simulink model "three_phase_full_bridge_rectification_mode"  (R2020b)
settings: Solver=VariableStepAuto  StartTime=0.0  StopTime=0.1  MaxStep=1e-3  RelTol=1e-3
libraries: powerlib x13, powerlib_meascontrol x4
settings Model: Creator=海王星之矛  LastModifiedBy=海王星之矛

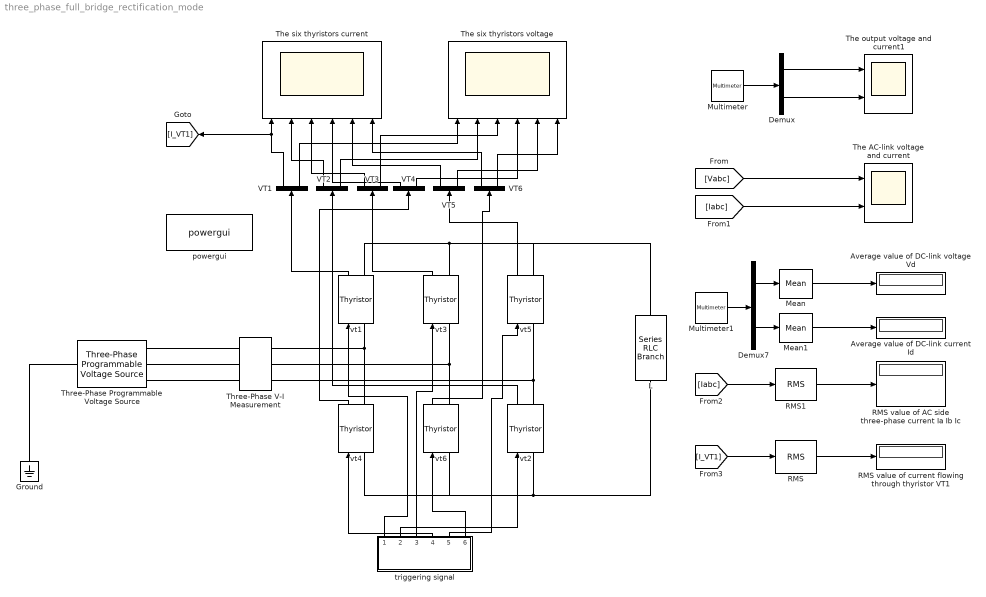
== system three_phase_full_bridge_rectification_mode ==
  Average value of DC-link current Id : Display
      settings: Decimation=2
  Average value of DC-link voltage Vd : Display
      settings: Decimation=2
  Demux : Demux  Outputs=2
  Demux7 : Demux  Outputs=2
  Ground : powerlib/Elements/Ground  LConnTagsString=a
  L : powerlib/Elements/Series RLC Branch  LConnTagsString=__new0  RConnTagsString=__new0  BranchType=RL  Resistance=1  Inductance=5e-3  SetiL0=on  InitialCurrent=0  Capacitance=1e-6  Setx0=off  InitialVoltage=0  Measurements=Branch voltage and current
  Mean : powerlib_meascontrol/Measurements/Mean  Freq=50  Vinit=0  Ts=0
  Mean1 : powerlib_meascontrol/Measurements/Mean  Freq=50  Vinit=0  Ts=0
  Multimeter : powerlib/Measurements/Multimeter  PhasorSimulation=off  OutputType=Complex  sel=[1 2]  L=2  Gain=[1 1]  yselected={'Ub: L','Ib: L'};  PSBOutputType=1  PSBequivalent=0  AxesSetting=[0,0.1,-100,100]  Display=0  SavedBlockNames=-11
  Multimeter1 : powerlib/Measurements/Multimeter  PhasorSimulation=off  OutputType=Complex  sel=[1 2]  L=2  Gain=[1 1]  yselected={'Ub: L','Ib: L'};  PSBOutputType=1  PSBequivalent=0  AxesSetting=[0,0.1,-100,100]  Display=0  SavedBlockNames=-11
  RMS : powerlib_meascontrol/Measurements/RMS  TrueRMS=on  Freq=60  RMSInit=120  Ts=0
  RMS value of AC side three-phase current Ia Ib Ic : Display
      settings: Decimation=2
  RMS value of current flowing through thyristor VT1 : Display
      settings: Decimation=2
  RMS1 : powerlib_meascontrol/Measurements/RMS  TrueRMS=on  Freq=60  RMSInit=120  Ts=0
  The AC-link voltage and current : Scope  NumInputPorts=2
  The output voltage and current1 : Scope  NumInputPorts=2
  The six thyristors current : Scope  NumInputPorts=6
  The six thyristors voltage : Scope  NumInputPorts=6
  Three-Phase Programmable Voltage Source : powerlib/Electrical Sources/Three-Phase Programmable Voltage Source  PositiveSequence="[220*sqrt(3)  0 50]"  VariationEntity=None  VariationType=Table of time-amplitude pairs  VariationTypeAlt=Step  VariationStep=0.5  VariationRate=10  VariationMagnitude=0.3  VariationFrequency=2  VariationTiming=[1 2]  VariationPhaseA=off  Amplitudes=[1 0.8 1.2 1.0]  TimeValues=[0 0.1 0.15 0.2]  HarmonicGeneration=off  HarmonicA=[3 0.2 -25 0]  HarmonicB=[2 0.15 35 2]  Timing="[0.05  3]"  BusType=swing  Pref=0  Qref=0  Qmin=-inf  Qmax=inf
  Three-Phase V-I Measurement : powerlib/Measurements/Three-Phase V-I Measurement  VoltageMeasurement=phase-to-ground  SetLabelV=on  LabelV=Vabc  Vpu=off  VpuLL=off  CurrentMeasurement=yes  SetLabelI=on  LabelI=Iabc  Ipu=off  Pbase=100e6  Vbase=500e3  OutputType=Complex  PhasorSimulation=off  PSBequivalent=0
  VT{1..6} (6 alike) : Demux  Outputs=2
  powergui : powerlib/powergui  Priority=1  SimulationMode=Continuous  SampleTime=50e-6  frequency=60  Iterations=50  frequencyindice=50  Pbase=100e6  ErrMax=1e-4  UnitsV=kV  UnitsW=MW  buscounter=0  FunctionMessages=off  echomessages=off  EnableUseOfTLC=off  CurrentSourceSwitches=off  DisableSnubberDevices=off  DisableRonSwitches=off  DisableVfSwitches=off  DisplayEquations=off  AutomaticDiscreteSolvers=off  SolverType=Tustin/Backward Euler (TBE)  Interpol=off  ExternalGateDelay=off  methode=off  Ts=100  x0status=blocks  SPID=on  SwTol=0  HookPort=off  NonlinearTolerance=1e-4  nMaxIteration=100  ContinueOnMaxIteration=off  RestoreLinks=warning  ResistiveCurrentMeasurement=off  Frange=[0:2:500]  Ylog=off  Xlog=on  ShowGrid=off  save=off  variable=ZData  structure=0  ZoomFFT=off  StartTime=0.0  cycles=1  DisplayStyle=1  fundamental=60  FreqAxis=off  MaxFrequency=1000  frequencyindicesteady=1  RmsSteady=1  display=off
  triggering signal : Subsystem  mask{alpha=85, width=50, higth=1}
  vt{1..6} (6 alike) : powerlib/Power Electronics/Thyristor  Ron=0.001  Lon=0  Vf=0.8  IC=0  Rs=500  Cs=250e-9  Measurements=on
  wires:
  triggering signal/1(Out1) -> vt1/1
  triggering signal/2(Out2) -> vt2/1
  triggering signal/3(Out3) -> vt3/1
  triggering signal/4(Out4) -> vt4/1
  triggering signal/5(Out5) -> vt5/1
  triggering signal/6(Out6) -> vt6/1
  Multimeter/1 -> Demux/1
  [Vabc] -> The AC-link voltage and current/1
  [Iabc] -> The AC-link voltage and current/2
  Demux/1 -> The output voltage and current1/1
  Demux/2 -> The output voltage and current1/2
  vt1/1 -> VT1/1
  vt2/1 -> VT2/1
  vt3/1 -> VT3/1
  vt4/1 -> VT4/1
  vt5/1 -> VT5/1
  vt6/1 -> VT6/1
  VT1/1 -> [I_VT1], The six thyristors current/1
  VT2/1 -> The six thyristors current/2
  VT3/1 -> The six thyristors current/3
  VT4/1 -> The six thyristors current/4
  VT5/1 -> The six thyristors current/5
  VT6/1 -> The six thyristors current/6
  VT1/2 -> The six thyristors voltage/1
  VT2/2 -> The six thyristors voltage/2
  VT3/2 -> The six thyristors voltage/3
  VT4/2 -> The six thyristors voltage/4
  VT5/2 -> The six thyristors voltage/5
  VT6/2 -> The six thyristors voltage/6
  Multimeter1/1 -> Demux7/1
  Demux7/1 -> Mean/1
  Demux7/2 -> Mean1/1
  Mean/1 -> Average value of DC-link voltage Vd/1
  Mean1/1 -> Average value of DC-link current Id/1
  [Iabc] -> RMS1/1
  RMS1/1 -> RMS value of AC side three-phase current Ia Ib Ic/1
  [I_VT1] -> RMS/1
  RMS/1 -> RMS value of current flowing through thyristor VT1/1
  connections:
  Ground/LConn1 -- Three-Phase Programmable Voltage Source/LConn1
  vt1/RConn1 -- L/LConn1 -- vt5/RConn1 -- vt3/RConn1
  vt6/RConn1 -- vt3/LConn1 -- Three-Phase V-I Measurement/RConn2
  vt2/RConn1 -- vt5/LConn1 -- Three-Phase V-I Measurement/RConn3
  L/RConn1 -- vt4/LConn1 -- vt6/LConn1 -- vt2/LConn1
  vt4/RConn1 -- vt1/LConn1 -- Three-Phase V-I Measurement/RConn1
  Three-Phase V-I Measurement/LConn1 -- Three-Phase Programmable Voltage Source/RConn1
  Three-Phase V-I Measurement/LConn2 -- Three-Phase Programmable Voltage Source/RConn2
  Three-Phase V-I Measurement/LConn3 -- Three-Phase Programmable Voltage Source/RConn3

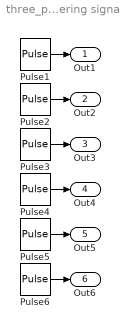
== system three_phase_full_bridge_rectification_mode/triggering signal ==
  Pulse1 : DiscretePulseGenerator  PulseType=Time based  Amplitude=higth  Period=1/50  PulseWidth=width  PhaseDelay=(30+alpha)/360*(1/50)
  Pulse2 : DiscretePulseGenerator  PulseType=Time based  Amplitude=higth  Period=1/50  PulseWidth=width  PhaseDelay=(90+alpha)/360*(1/50)
  Pulse3 : DiscretePulseGenerator  PulseType=Time based  Amplitude=higth  Period=1/50  PulseWidth=width  PhaseDelay=(150+alpha)/360*(1/50)
  Pulse4 : DiscretePulseGenerator  PulseType=Time based  Amplitude=higth  Period=1/50  PulseWidth=width  PhaseDelay=(210+alpha)/360*(1/50)
  Pulse5 : DiscretePulseGenerator  PulseType=Time based  Amplitude=higth  Period=1/50  PulseWidth=width  PhaseDelay=(270+alpha)/360*(1/50)
  Pulse6 : DiscretePulseGenerator  PulseType=Time based  Amplitude=higth  Period=1/50  PulseWidth=width  PhaseDelay=(330+alpha)/360*(1/50)
  Out1 : Outport
  Out2 : Outport  Port=2
  Out3 : Outport  Port=3
  Out4 : Outport  Port=4
  Out5 : Outport  Port=5
  Out6 : Outport  Port=6
  wires:
  Pulse1/1 -> Out1/1
  Pulse2/1 -> Out2/1
  Pulse3/1 -> Out3/1
  Pulse4/1 -> Out4/1
  Pulse5/1 -> Out5/1
  Pulse6/1 -> Out6/1
